simulink model "Saturator"  (R2018b)
settings: Solver=VariableStepAuto  StartTime=0.0  StopTime=10.0  RelTol=1e-3
settings Model: Creator=mhosue  LastModifiedBy=mhosue

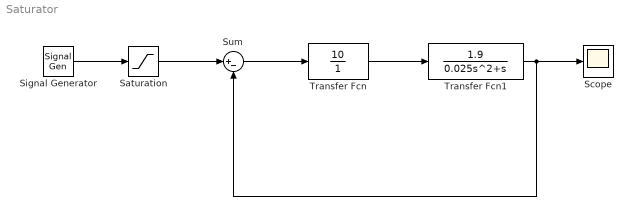
== system Saturator ==
  Saturation : Saturate  UpperLimit=0.7  LowerLimit=-0.7
  Scope : Scope
  Signal Generator : SignalGenerator  Units=rad/sec
  Sum : Sum  Inputs=|+-
  Transfer Fcn : TransferFcn  Numerator=[10]  Denominator=[1]
  Transfer Fcn1 : TransferFcn  Numerator=[1.9]  Denominator=[0.025 1 0]
  wires:
  Transfer Fcn/1 -> Transfer Fcn1/1
  Sum/1 -> Transfer Fcn/1
  Transfer Fcn1/1 -> Scope/1, Sum/2
  Saturation/1 -> Sum/1
  Signal Generator/1 -> Saturation/1
